simulink model "simulation"  (R2024a)
settings: Solver=FixedStepAuto  StartTime=0.0  StopTime=15  FixedStep=0.001  RelTol=1e-3
InitFcn:
  | clear all
  | clc
  | 
  | %% Modell Parameter Drosselklappe
  | Phi_LHP = 0;
  | R = 2.0;
  | Cm = 4.19*exp(-3);
  | L = 20*exp(-6);
  | J = 1.7*exp(-6);
  | Cf = 2.2*exp(-4);
  | D = 1*exp(-7);
  | Mfr = 1*exp(-6);
  | Mpre = 1*exp(-6);
  | 
  | %% Reglerparameter PI-Regler
  | Kp = 1;
  | Ki = 0.1;
settings Model: Creator=danie  LastModifiedBy=danie

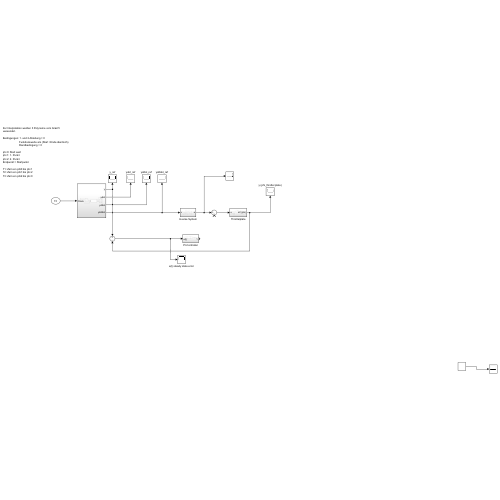
[thumbnail: Simulink's stored preview of the top-level diagram]
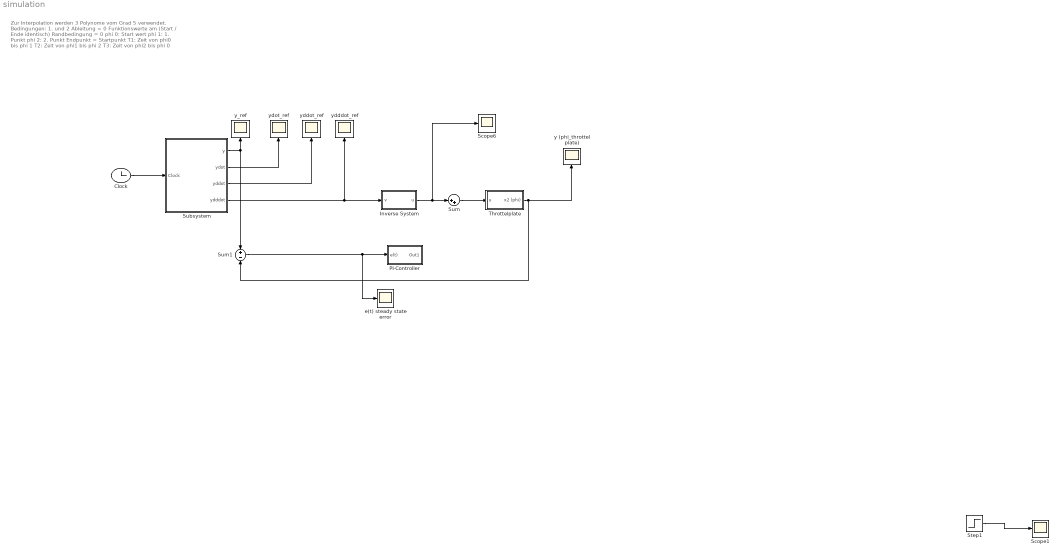
== system simulation ==
  note: Zur Interpolation werden 3 Polynome vom Grad 5 verwendet.
      |
      | Bedingungen: 1. und 2 Ableitung = 0
      | 			 Funktionswerte am (Start / Ende identisch)
      | 			 Randbedingung = 0
      |
      | phi 0: Start wert
      | phi 1: 1. Punkt
      | phi 2: 2. Punkt
      | Endpunkt = Startpunkt
      |
      | T1: Zeit von phi0 bis phi 1
      | T2: Zeit von phi1 bis phi 2
      | T3: Zeit von phi2 bis phi 0
  Clock : Clock
  Inverse System : Subsystem
  PI-Controller : Subsystem
  Scope1 : Scope
  Scope6 : Scope
  Step1 : Step  SampleTime=0
  Subsystem : Subsystem
  Sum : Sum  Inputs=|++
  Sum1 : Sum  Inputs=+|-
  Throttelplate : Subsystem
  e(t) steady state error : Scope
  y (phi_throttel plate) : Scope
  y_ref : Scope
  ydddot_ref : Scope
  yddot_ref : Scope
  ydot_ref : Scope
  wires:
  Step1/1 -> Scope1/1
  Throttelplate/1(x2 (phi)) -> Sum1/2, y (phi_throttel plate)/1
  Clock/1 -> Subsystem/1(Clock)
  Sum/1 -> Throttelplate/1(u)
  Inverse System/1(u) -> Scope6/1, Sum/1
  Sum1/1 -> e(t) steady state error/1, PI-Controller/1(e(t))
  Subsystem/4(ydddot) -> Inverse System/1(v), ydddot_ref/1
  Subsystem/1(y) -> Sum1/1, y_ref/1
  Subsystem/2(ydot) -> ydot_ref/1
  Subsystem/3(yddot) -> yddot_ref/1

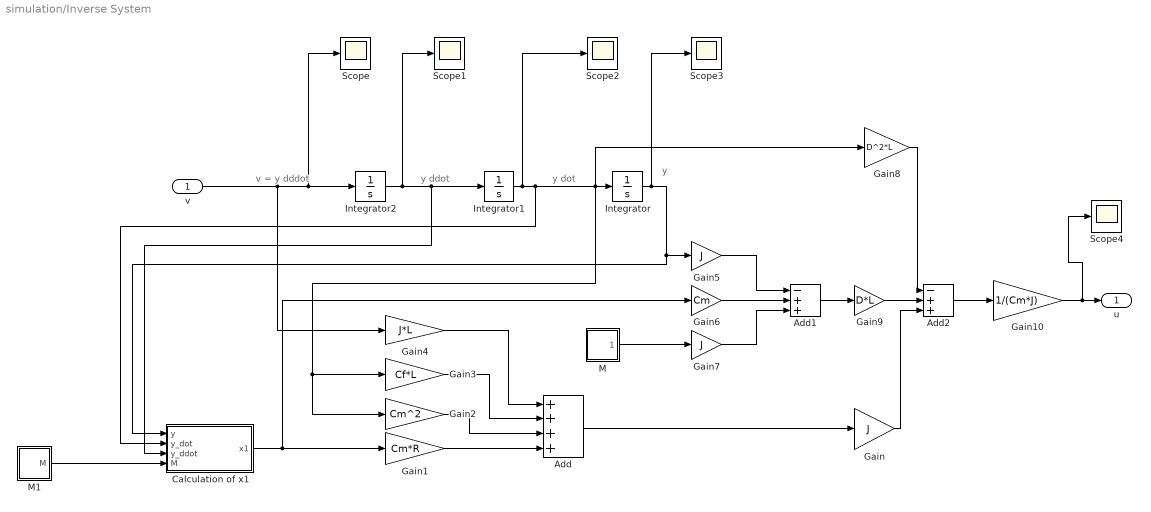
== system simulation/Inverse System ==
  note: v = y dddot
  note: y ddot
  note: y dot
  note: y
  v : Inport
  Add : Sum  Inputs=++++
  Add1 : Sum  Inputs=-++
  Add2 : Sum  Inputs=-++
  Calculation of x1 : Subsystem
  Gain : Gain  Gain=J
  Gain1 : Gain  Gain=Cm*R
  Gain10 : Gain  Gain=1/(Cm*J)
  Gain2 : Gain  Gain=Cm^2
  Gain3 : Gain  Gain=Cf*L
  Gain4 : Gain  Gain=J*L
  Gain5 : Gain  Gain=J
  Gain6 : Gain  Gain=Cm
  Gain7 : Gain  Gain=J
  Gain8 : Gain  Gain=D^2*L
  Gain9 : Gain  Gain=D*L
  Integrator : Integrator
  Integrator1 : Integrator
  Integrator2 : Integrator
  M : Subsystem
  M1 : Subsystem
  Scope{,1..4} (5 alike) : Scope
  u : Outport
  wires:
  Integrator1/1 -> Scope2/1, Calculation of x1/2(y_dot), Gain8/1, Gain2/1, Gain3/1, Integrator/1
  Integrator2/1 -> Scope1/1, Calculation of x1/3(y_ddot), Integrator1/1
  Integrator/1 -> Scope3/1, Calculation of x1/1(y), Gain5/1
  v/1 -> Scope/1, Integrator2/1, Gain4/1
  Add/1 -> Gain/1
  Gain1/1 -> Add/4
  Gain2/1 -> Add/3
  Gain3/1 -> Add/2
  Gain4/1 -> Add/1
  M/1(Out1) -> Gain7/1
  Gain7/1 -> Add1/3
  Gain6/1 -> Add1/2
  Gain5/1 -> Add1/1
  Add1/1 -> Gain9/1
  Gain10/1 -> Scope4/1, u/1
  Add2/1 -> Gain10/1
  Gain/1 -> Add2/3
  Gain9/1 -> Add2/2
  Gain8/1 -> Add2/1
  Calculation of x1/1(x1) -> Gain6/1, Gain1/1
  M1/1(M) -> Calculation of x1/4(M)

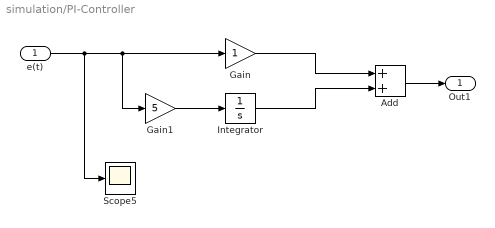
== system simulation/PI-Controller ==
  e(t) : Inport
  Add : Sum
  Gain : Gain
  Gain1 : Gain  Gain=5
  Integrator : Integrator
  Scope5 : Scope
  Out1 : Outport
  wires:
  Add/1 -> Out1/1
  e(t)/1 -> Scope5/1, Gain1/1, Gain/1
  Gain/1 -> Add/1
  Integrator/1 -> Add/2
  Gain1/1 -> Integrator/1

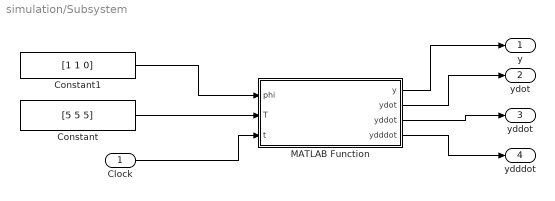
== system simulation/Subsystem ==
  Clock : Inport
  Constant : Constant  Value=[5 5 5]  VectorParams1D=off
  Constant1 : Constant  Value=[1 1 0]
  MATLAB Function : MATLAB Function  TreatAsAtomicUnit=on
  y : Outport
  ydot : Outport  Port=2
  yddot : Outport  Port=3
  ydddot : Outport  Port=4
  wires:
  MATLAB Function/1(y) -> y/1
  MATLAB Function/2(ydot) -> ydot/1
  MATLAB Function/3(yddot) -> yddot/1
  MATLAB Function/4(ydddot) -> ydddot/1
  Clock/1 -> MATLAB Function/3(t)
  Constant/1 -> MATLAB Function/2(T)
  Constant1/1 -> MATLAB Function/1(phi)

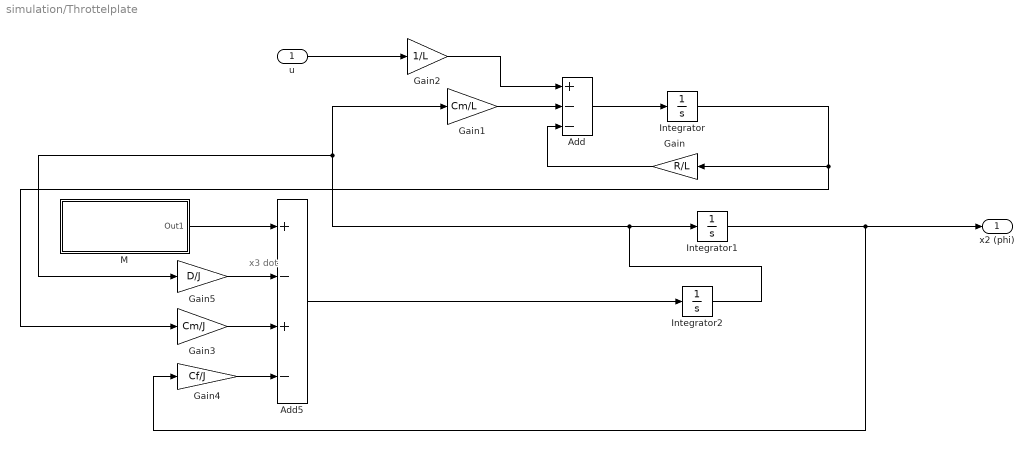
== system simulation/Throttelplate ==
  note: x3 dot
  u : Inport
  Add : Sum  Inputs=+--
  Add5 : Sum  Inputs=+-+-
  Gain : Gain  Gain=R/L
  Gain1 : Gain  Gain=Cm/L
  Gain2 : Gain  Gain=1/L
  Gain3 : Gain  Gain=Cm/J
  Gain4 : Gain  Gain=Cf/J
  Gain5 : Gain  Gain=D/J
  Integrator : Integrator
  Integrator1 : Integrator
  Integrator2 : Integrator
  M : Subsystem
  x2 (phi) : Outport
  wires:
  Integrator/1 -> Gain/1, Gain3/1
  Add/1 -> Integrator/1
  u/1 -> Gain2/1
  Integrator1/1 -> Gain4/1, x2 (phi)/1
  Gain2/1 -> Add/1
  Gain/1 -> Add/3
  Gain1/1 -> Add/2
  Integrator2/1 -> Gain5/1, Gain1/1, Integrator1/1
  Add5/1 -> Integrator2/1
  Gain5/1 -> Add5/2
  M/1(Out1) -> Add5/1
  Gain3/1 -> Add5/3
  Gain4/1 -> Add5/4

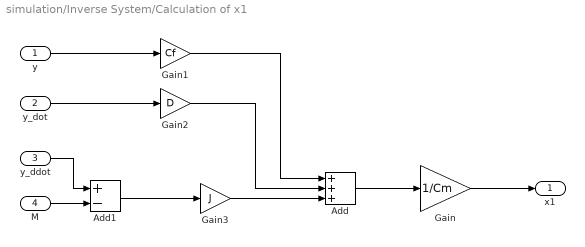
== system simulation/Inverse System/Calculation of x1 ==
  y : Inport
  y_dot : Inport  Port=2
  y_ddot : Inport  Port=3
  M : Inport  Port=4
  Add : Sum  Inputs=+++
  Add1 : Sum  Inputs=+-
  Gain : Gain  Gain=1/Cm
  Gain1 : Gain  Gain=Cf
  Gain2 : Gain  Gain=D
  Gain3 : Gain  Gain=J
  x1 : Outport
  wires:
  Add/1 -> Gain/1
  Gain/1 -> x1/1
  y/1 -> Gain1/1
  Gain1/1 -> Add/1
  y_dot/1 -> Gain2/1
  Gain2/1 -> Add/2
  y_ddot/1 -> Add1/1
  Add1/1 -> Gain3/1
  Gain3/1 -> Add/3
  M/1 -> Add1/2

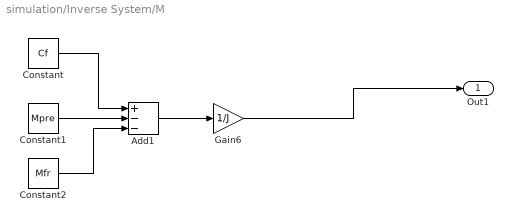
== system simulation/Inverse System/M ==
  Add1 : Sum  Inputs=+--
  Constant : Constant  Value=Cf
  Constant1 : Constant  Value=Mpre
  Constant2 : Constant  Value=Mfr
  Gain6 : Gain  Gain=1/J
  Out1 : Outport
  wires:
  Constant/1 -> Add1/1
  Add1/1 -> Gain6/1
  Constant2/1 -> Add1/3
  Constant1/1 -> Add1/2
  Gain6/1 -> Out1/1

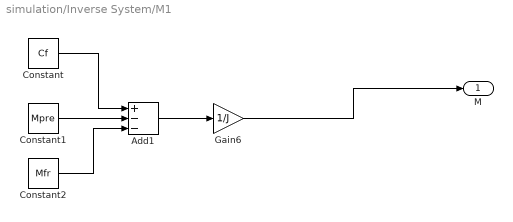
== system simulation/Inverse System/M1 ==
  Add1 : Sum  Inputs=+--
  Constant : Constant  Value=Cf
  Constant1 : Constant  Value=Mpre
  Constant2 : Constant  Value=Mfr
  Gain6 : Gain  Gain=1/J
  M : Outport
  wires:
  Constant/1 -> Add1/1
  Add1/1 -> Gain6/1
  Constant2/1 -> Add1/3
  Constant1/1 -> Add1/2
  Gain6/1 -> M/1

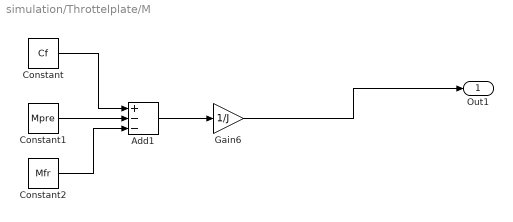
== system simulation/Throttelplate/M ==
  Add1 : Sum  Inputs=+--
  Constant : Constant  Value=Cf
  Constant1 : Constant  Value=Mpre
  Constant2 : Constant  Value=Mfr
  Gain6 : Gain  Gain=1/J
  Out1 : Outport
  wires:
  Constant/1 -> Add1/1
  Add1/1 -> Gain6/1
  Constant2/1 -> Add1/3
  Constant1/1 -> Add1/2
  Gain6/1 -> Out1/1

== matlab function simulation/Subsystem/MATLAB Function ==
  data: phi input; y output; T input; t input; ydot output; yddot output; ydddot output
function [y, ydot, yddot, ydddot] = fcn(phi, T, t)
   
    % Gesamtzeit aller Intervalle
    total_duration = sum(T);
    
    % Modulo-Operation, um t zyklisch zu machen
    t_mod = mod(t, total_duration);

    t_start = 0; % Init start time
    
    % Durchlaufe alle Intervalle
    for i = 1:length(T)
        % Bestimme das aktuelle Intervall
        t_end = t_start + T(i);
        
        % Prüfe, ob t_mod in das aktuelle Intervall fällt
        if t_mod < t_end
            % Evaluiere das entsprechende Polynom
            if i <= 1
                coeffs = compute_coeffs(0, phi(i), T(i));
            else
                coeffs = compute_coeffs(phi(i-1), phi(i), T(i));
            end    
            % Berechnung der Koeffizienten der Ableitungen
            coeffs_first_derivative  = polyder(coeffs);
            coeffs_second_derivative = polyder(coeffs_first_derivative); 
            coeffs_third_derivative  = polyder(coeffs_second_derivative); % dritte Ableitung
            % Auswertung zum Zeitpunkt t (eval_time)
            y      = polyval(coeffs, t_mod - t_start);
            ydot   = polyval(coeffs_first_derivative, t_mod - t_start);
            yddot  = polyval(coeffs_second_derivative, t_mod - t_start);
            ydddot = polyval(coeffs_third_derivative, t_mod - t_start);
            return;
        end
        
        % Aktualisiere den Startzeitpunkt für das nächste Intervall
        t_start = t_end;
    end

    % FEHLER FALL
    y      = 0;
    ydot   = 0;
    yddot  = 0;
    ydddot = 0;
    

end

function coeffs = compute_coeffs(phi_0, phi_d, T)
    % Matrix A
    A = [0 0 0 0 0 1;
         T^5 T^4 T^3 T^2 T 1;
         0 0 0 2 0 0;
         0 0 0 0 1 0;
         5*T^4 4*T^3 3*T^2 2*T 1 0;
         20*T^3 12*T^2 2*T 1 0 0];
    
    % Vector b
    b = transpose([phi_0 phi_d 0 0 0 0]);

    % Berechnung der Koeffizienten
    coeffs = A\b;
end
